simulink model "hw4_p4_pitchAttitude_control"  (R2020a)
settings: Solver=VariableStepAuto  StartTime=0.0  StopTime=10.0  RelTol=1e-3
undefined symbols (not defined in the file or in its folder): init, Kp, Krg
settings Model: Creator=Tomo  LastModifiedBy=Tomo

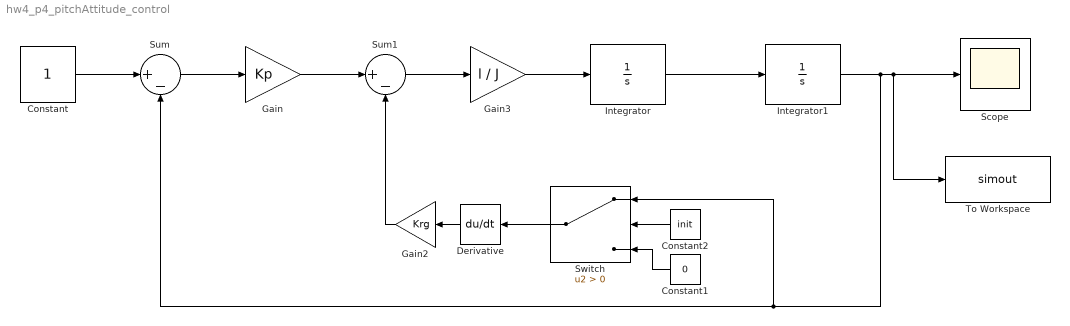
== system hw4_p4_pitchAttitude_control ==
  Constant : Constant
  Constant1 : Constant  Value=0
  Constant2 : Constant  Value=init
  Derivative : Derivative
  Gain : Gain  Gain=Kp
  Gain2 : Gain  Gain=Krg
  Gain3 : Gain  Gain=l / J
  Integrator : Integrator
  Integrator1 : Integrator
  Scope : Scope
  Sum : Sum  Inputs=|+-
  Sum1 : Sum  Inputs=|+-
  Switch : Switch  Criteria=u2 > Threshold
  To Workspace : ToWorkspace  VariableName=simout  SaveFormat=Timeseries  SampleTime=-1
  wires:
  Constant/1 -> Sum/1
  Sum/1 -> Gain/1
  Gain/1 -> Sum1/1
  Sum1/1 -> Gain3/1
  Integrator/1 -> Integrator1/1
  Integrator1/1 -> Switch/1, Sum/2, To Workspace/1, Scope/1
  Derivative/1 -> Gain2/1
  Gain2/1 -> Sum1/2
  Switch/1 -> Derivative/1
  Constant1/1 -> Switch/3
  Constant2/1 -> Switch/2
  Gain3/1 -> Integrator/1
